simulink model "Sim1_3_2_simu"  (R2021a)
settings: Solver=VariableStepAuto  StartTime=0.0  StopTime=Ts*1e6  RelTol=1e-3
values from neighbouring files (symbols this model uses):
  sysd = c2d(G, Ts, 'zoh')    [Sim1_1.m]    (also in Sim1_2.m; Sim1_2_5.m; Sim1_2_CovRes_Fast.m; Sim1_2_CovRes_Slow.m)
  Ts = (2*pi)/(20*bw)    [Sim1_1.m]    (also in Sim1_2.m; Sim1_2_5.m; Sim1_2_CovRes_Fast.m; Sim1_2_CovRes_Slow.m)
undefined symbols (not defined in the file or in its folder): C
libraries: simulink x2
settings Model: Creator=ASUS  LastModifiedBy=ASUS

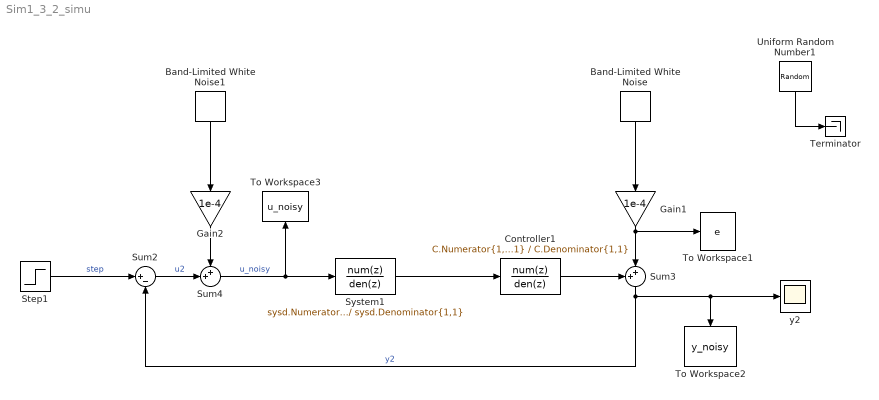
== system Sim1_3_2_simu ==
  Band-Limited White Noise : simulink/Sources/Band-Limited White Noise  Cov=[0.01]  Ts=Ts  seed=[23341]
  Band-Limited White Noise1 : simulink/Sources/Band-Limited White Noise  Cov=[0.01]  Ts=Ts  seed=[23342]
  Controller1 : DiscreteTransferFcn  Numerator=C.Numerator{1,1}  Denominator=C.Denominator{1,1}
  Gain1 : Gain  Gain=1e-4
  Gain2 : Gain  Gain=1e-4
  Step1 : Step  Time=0  After=5  SampleTime=0
  Sum2 : Sum  Inputs=|+-
  Sum3 : Sum  Inputs=++|
  Sum4 : Sum  Inputs=++|
  System1 : DiscreteTransferFcn  Numerator=sysd.Numerator{1,1}  Denominator=sysd.Denominator{1,1}
  Terminator : Terminator
  To Workspace1 : ToWorkspace  VariableName=e  SampleTime=-1
  To Workspace2 : ToWorkspace  VariableName=y_noisy  SampleTime=-1
  To Workspace3 : ToWorkspace  VariableName=u_noisy  SampleTime=-1
  Uniform Random Number1 : UniformRandomNumber  SampleTime=Ts
  y2 : Scope
  wires:
  Gain2/1 -> Sum4/1
  Band-Limited White Noise1/1 -> Gain2/1
  Sum3/1 -> Sum2/2, y2/1, To Workspace2/1  "y2"
  Gain1/1 -> Sum3/2, To Workspace1/1
  System1/1 -> Controller1/1
  Controller1/1 -> Sum3/1
  Sum2/1 -> Sum4/2  "u2"
  Sum4/1 -> To Workspace3/1, System1/1  "u_noisy"
  Step1/1 -> Sum2/1  "step"
  Uniform Random Number1/1 -> Terminator/1
  Band-Limited White Noise/1 -> Gain1/1
